simulink model "speed_rpm_indicator"  (R2020b)
settings: Solver=VariableStepAuto  StartTime=0.0  StopTime=10.0  RelTol=1e-3
settings Model: Creator=Training  LastModifiedBy=Training

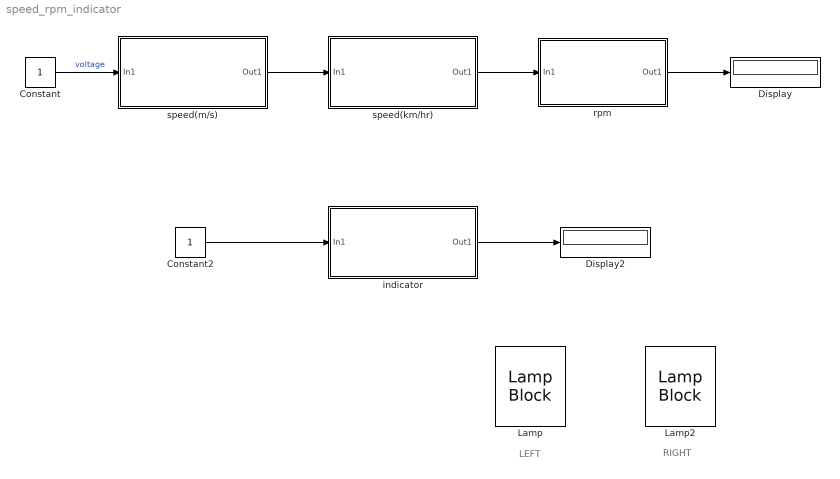
== system speed_rpm_indicator ==
  note: LEFT
  note: RIGHT
  Constant : Constant
  Constant2 : Constant
  Display : Display
  Display2 : Display
  Lamp : LampBlock
  Lamp2 : LampBlock
  indicator : Subsystem
  rpm : Subsystem
  speed(km/hr) : Subsystem
  speed(m/s) : Subsystem
  wires:
  rpm/1(Out1) -> Display/1
  speed(m/s)/1(Out1) -> speed(km/hr)/1(In1)
  Constant/1 -> speed(m/s)/1(In1)  "voltage"
  speed(km/hr)/1(Out1) -> rpm/1(In1)
  indicator/1(Out1) -> Display2/1
  Constant2/1 -> indicator/1(In1)

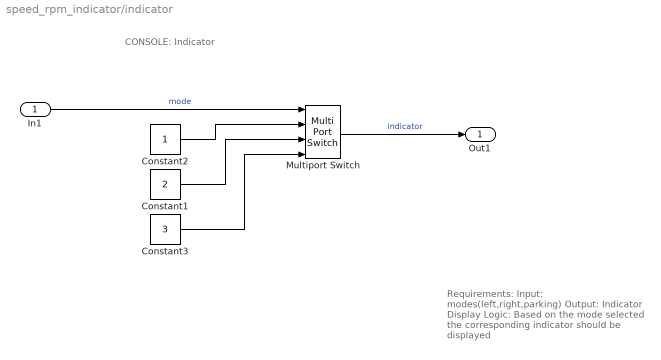
== system speed_rpm_indicator/indicator ==
  note: CONSOLE: Indicator
  note: Requirements:
      | Input: modes(left,right,parking)
      | Output: Indicator Display
      | Logic: Based on the mode selected the corresponding indicator should be displayed
  In1 : Inport
  Constant1 : Constant  Value=2
  Constant2 : Constant
  Constant3 : Constant  Value=3
  Multiport Switch : MultiPortSwitch
  Out1 : Outport
  wires:
  In1/1 -> Multiport Switch/1  "mode"
  Multiport Switch/1 -> Out1/1  "indicator"
  Constant2/1 -> Multiport Switch/2
  Constant1/1 -> Multiport Switch/3
  Constant3/1 -> Multiport Switch/4

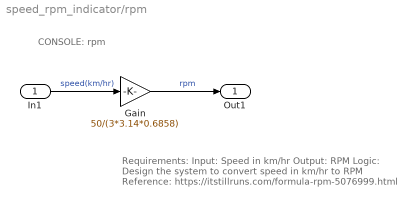
== system speed_rpm_indicator/rpm ==
  note: CONSOLE: rpm
  note: Requirements:
      | Input: Speed in km/hr
      | Output: RPM
      | Logic: Design the system to convert speed in km/hr to RPM Reference: https://itstillruns.com/formula-rpm-5076999.html
  In1 : Inport
  Gain : Gain  Gain=50/(3*3.14*0.6858)
  Out1 : Outport
  wires:
  In1/1 -> Gain/1  "speed(km/hr)"
  Gain/1 -> Out1/1  "rpm"

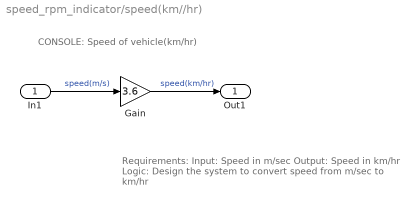
== system speed_rpm_indicator/speed(km//hr) ==
  note: CONSOLE: Speed of vehicle(km/hr)
  note: Requirements:
      | Input: Speed in m/sec
      | Output: Speed in km/hr
      | Logic: Design the system to convert speed from m/sec to km/hr
  In1 : Inport
  Gain : Gain  Gain=3.6
  Out1 : Outport
  wires:
  In1/1 -> Gain/1  "speed(m/s)"
  Gain/1 -> Out1/1  "speed(km/hr)"

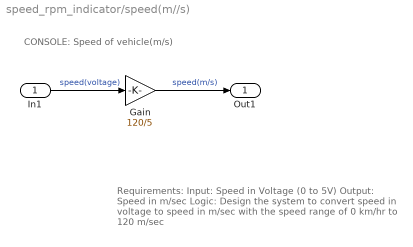
== system speed_rpm_indicator/speed(m//s) ==
  note: CONSOLE: Speed of vehicle(m/s)
  note: Requirements:
      | Input: Speed in Voltage (0 to 5V)
      | Output: Speed in m/sec
      | Logic: Design the system to convert speed in voltage to
      | speed in m/sec with the speed range of 0 km/hr to 120 m/sec
  In1 : Inport
  Gain : Gain  Gain=120/5
  Out1 : Outport
  wires:
  In1/1 -> Gain/1  "speed(voltage)"
  Gain/1 -> Out1/1  "speed(m/s)"
